simulink model "Casc_Filter_x4"  (Simulink 6.4)
settings: Solver=ode45  StartTime=0.0  StopTime=4100/sampling_freq  RelTol=1e-3
undefined symbols (not defined in the file): A, B, filter_clk, Fs, get, h_g, h_k, PCIN, sampling_freq
libraries: xbsIndex_r4 x851, dspsnks4 x9, simulink x2, dspsrcs4 x1
(part 8 of 8)

== system Casc_Filter_x4/DDC/DDC B/Gaussian FIR Filters/Gaussian FIR Filter1/Symmetric Data Flow/Symmetric Shift Register ==
  Shift In 1 : Inport
  Counter : Inport  Port=2
  Counter Inv : Inport  Port=3
  Shift In 2 : Inport  Port=4
  ASR : xbsIndex_r4/Addressable Shift Register  infer_latency=off  depth=12  initVector=[0]  en=off  dbl_ovrd=off  use_behavioral_HDL=off  use_rpm=off  block_type=addrsr
      settings: infoedit="Delay of  configurable length.  Any element  in the delay     line   can    be   addressed   and   driven    onto   the   output     port.<P><P>Hardware  notes: Implemented  using SRL16s.     If Virtex-4, Virtex-II or Spartan-3 devices are used, multiple SRLC16s are cascaded together."  xl_area=[9 0 0 18 0 0 0]  block_version=VER_STRING_GOES_HERE
  ASR1 : xbsIndex_r4/Addressable Shift Register  infer_latency=off  depth=12  initVector=[0]  en=off  dbl_ovrd=off  use_behavioral_HDL=off  use_rpm=off  block_type=addrsr
      settings: infoedit="Delay of  configurable length.  Any element  in the delay     line   can    be   addressed   and   driven    onto   the   output     port.<P><P>Hardware  notes: Implemented  using SRL16s.     If Virtex-4, Virtex-II or Spartan-3 devices are used, multiple SRLC16s are cascaded together."  xl_area=[9 0 0 18 0 0 0]  block_version=VER_STRING_GOES_HERE
  AddSub : xbsIndex_r4/AddSub  mode=Addition  use_carryin=off  use_carryout=off  en=off  latency=1  precision=User Defined  arith_type="Signed  (2's comp)"  n_bits=18  bin_pt=16  quantization="Round  (unbiased: +/- Inf)"  overflow=Saturate  dbl_ovrd=off  use_behavioral_HDL=off  pipelined=on  use_rpm=on  block_type=addsub
      settings: xl_area=[19 0 0 37 0 0 0]  block_version=VER_STRING_GOES_HERE
  Delay : xbsIndex_r4/Delay  en=off  latency=12  dbl_ovrd=off  reg_retiming=off  block_type=delay
      settings: infoedit=Hardware notes: A delay line is a chain, each link of which is an SRL16 followed by a flip-flop. If register retiming is enabled, the delay line is a chain of flip-flops.  xl_area=[9 18 0 18 0 0 0]  block_version=VER_STRING_GOES_HERE
  Delay1 : xbsIndex_r4/Delay  en=off  latency=12  dbl_ovrd=off  reg_retiming=off  block_type=delay
      settings: infoedit=Hardware notes: A delay line is a chain, each link of which is an SRL16 followed by a flip-flop. If register retiming is enabled, the delay line is a chain of flip-flops.  xl_area=[9 18 0 18 0 0 0]  block_version=VER_STRING_GOES_HERE
  Register : xbsIndex_r4/Register  init=0  rst=off  en=off  dbl_ovrd=off  block_type=register
      settings: block_version=8.2
  Register1 : xbsIndex_r4/Register  init=0  rst=off  en=off  dbl_ovrd=off  block_type=register
      settings: block_version=8.2
  Shift Out 1 : Outport
  Sum Out : Outport  Port=2
  Shift Out 2 : Outport  Port=3
  wires:
  Counter Inv/1 -> ASR1/2
  Shift In 1/1 -> ASR/1, Delay/1
  Shift In 2/1 -> Delay1/1, ASR1/1
  Counter/1 -> ASR/2
  ASR/1 -> Register/1
  ASR1/1 -> Register1/1
  AddSub/1 -> Sum Out/1
  Delay1/1 -> Shift Out 2/1
  Delay/1 -> Shift Out 1/1
  Register/1 -> AddSub/1
  Register1/1 -> AddSub/2

== system Casc_Filter_x4/DDC/DDC B/Gaussian FIR Filters/Gaussian FIR Filter1/Symmetric Data Flow/Symmetric Shift Register1 ==
  Shift In 1 : Inport
  Counter : Inport  Port=2
  Counter Inv : Inport  Port=3
  Shift In 2 : Inport  Port=4
  ASR : xbsIndex_r4/Addressable Shift Register  infer_latency=off  depth=12  initVector=[0]  en=off  dbl_ovrd=off  use_behavioral_HDL=off  use_rpm=off  block_type=addrsr
      settings: infoedit="Delay of  configurable length.  Any element  in the delay     line   can    be   addressed   and   driven    onto   the   output     port.<P><P>Hardware  notes: Implemented  using SRL16s.     If Virtex-4, Virtex-II or Spartan-3 devices are used, multiple SRLC16s are cascaded together."  xl_area=[9 0 0 18 0 0 0]  block_version=VER_STRING_GOES_HERE
  ASR1 : xbsIndex_r4/Addressable Shift Register  infer_latency=off  depth=12  initVector=[0]  en=off  dbl_ovrd=off  use_behavioral_HDL=off  use_rpm=off  block_type=addrsr
      settings: infoedit="Delay of  configurable length.  Any element  in the delay     line   can    be   addressed   and   driven    onto   the   output     port.<P><P>Hardware  notes: Implemented  using SRL16s.     If Virtex-4, Virtex-II or Spartan-3 devices are used, multiple SRLC16s are cascaded together."  xl_area=[9 0 0 18 0 0 0]  block_version=VER_STRING_GOES_HERE
  AddSub : xbsIndex_r4/AddSub  mode=Addition  use_carryin=off  use_carryout=off  en=off  latency=1  precision=User Defined  arith_type="Signed  (2's comp)"  n_bits=18  bin_pt=16  quantization="Round  (unbiased: +/- Inf)"  overflow=Saturate  dbl_ovrd=off  use_behavioral_HDL=off  pipelined=on  use_rpm=on  block_type=addsub
      settings: xl_area=[19 0 0 37 0 0 0]  block_version=VER_STRING_GOES_HERE
  Delay : xbsIndex_r4/Delay  en=off  latency=12  dbl_ovrd=off  reg_retiming=off  block_type=delay
      settings: infoedit=Hardware notes: A delay line is a chain, each link of which is an SRL16 followed by a flip-flop. If register retiming is enabled, the delay line is a chain of flip-flops.  xl_area=[9 18 0 18 0 0 0]  block_version=VER_STRING_GOES_HERE
  Delay1 : xbsIndex_r4/Delay  en=off  latency=12  dbl_ovrd=off  reg_retiming=off  block_type=delay
      settings: infoedit=Hardware notes: A delay line is a chain, each link of which is an SRL16 followed by a flip-flop. If register retiming is enabled, the delay line is a chain of flip-flops.  xl_area=[9 18 0 18 0 0 0]  block_version=VER_STRING_GOES_HERE
  Register : xbsIndex_r4/Register  init=0  rst=off  en=off  dbl_ovrd=off  block_type=register
      settings: block_version=8.2
  Register1 : xbsIndex_r4/Register  init=0  rst=off  en=off  dbl_ovrd=off  block_type=register
      settings: block_version=8.2
  Shift Out 1 : Outport
  Sum Out : Outport  Port=2
  Shift Out 2 : Outport  Port=3
  wires:
  Counter Inv/1 -> ASR1/2
  Shift In 1/1 -> ASR/1, Delay/1
  Shift In 2/1 -> Delay1/1, ASR1/1
  Counter/1 -> ASR/2
  ASR/1 -> Register/1
  ASR1/1 -> Register1/1
  AddSub/1 -> Sum Out/1
  Delay1/1 -> Shift Out 2/1
  Delay/1 -> Shift Out 1/1
  Register/1 -> AddSub/1
  Register1/1 -> AddSub/2

== system Casc_Filter_x4/DDC/DDC B/Gaussian FIR Filters/Gaussian FIR Filter1/Symmetric Data Flow/Symmetric Shift Register2 ==
  Shift In 1 : Inport
  Counter : Inport  Port=2
  Counter Inv : Inport  Port=3
  Shift In 2 : Inport  Port=4
  ASR : xbsIndex_r4/Addressable Shift Register  infer_latency=off  depth=12  initVector=[0]  en=off  dbl_ovrd=off  use_behavioral_HDL=off  use_rpm=off  block_type=addrsr
      settings: infoedit="Delay of  configurable length.  Any element  in the delay     line   can    be   addressed   and   driven    onto   the   output     port.<P><P>Hardware  notes: Implemented  using SRL16s.     If Virtex-4, Virtex-II or Spartan-3 devices are used, multiple SRLC16s are cascaded together."  xl_area=[9 0 0 18 0 0 0]  block_version=VER_STRING_GOES_HERE
  ASR1 : xbsIndex_r4/Addressable Shift Register  infer_latency=off  depth=12  initVector=[0]  en=off  dbl_ovrd=off  use_behavioral_HDL=off  use_rpm=off  block_type=addrsr
      settings: infoedit="Delay of  configurable length.  Any element  in the delay     line   can    be   addressed   and   driven    onto   the   output     port.<P><P>Hardware  notes: Implemented  using SRL16s.     If Virtex-4, Virtex-II or Spartan-3 devices are used, multiple SRLC16s are cascaded together."  xl_area=[9 0 0 18 0 0 0]  block_version=VER_STRING_GOES_HERE
  AddSub : xbsIndex_r4/AddSub  mode=Addition  use_carryin=off  use_carryout=off  en=off  latency=1  precision=User Defined  arith_type="Signed  (2's comp)"  n_bits=18  bin_pt=16  quantization="Round  (unbiased: +/- Inf)"  overflow=Saturate  dbl_ovrd=off  use_behavioral_HDL=off  pipelined=on  use_rpm=on  block_type=addsub
      settings: xl_area=[19 0 0 37 0 0 0]  block_version=VER_STRING_GOES_HERE
  Delay : xbsIndex_r4/Delay  en=off  latency=12  dbl_ovrd=off  reg_retiming=off  block_type=delay
      settings: infoedit=Hardware notes: A delay line is a chain, each link of which is an SRL16 followed by a flip-flop. If register retiming is enabled, the delay line is a chain of flip-flops.  xl_area=[9 18 0 18 0 0 0]  block_version=VER_STRING_GOES_HERE
  Delay1 : xbsIndex_r4/Delay  en=off  latency=12  dbl_ovrd=off  reg_retiming=off  block_type=delay
      settings: infoedit=Hardware notes: A delay line is a chain, each link of which is an SRL16 followed by a flip-flop. If register retiming is enabled, the delay line is a chain of flip-flops.  xl_area=[9 18 0 18 0 0 0]  block_version=VER_STRING_GOES_HERE
  Register : xbsIndex_r4/Register  init=0  rst=off  en=off  dbl_ovrd=off  block_type=register
      settings: block_version=8.2
  Register1 : xbsIndex_r4/Register  init=0  rst=off  en=off  dbl_ovrd=off  block_type=register
      settings: block_version=8.2
  Shift Out 1 : Outport
  Sum Out : Outport  Port=2
  Shift Out 2 : Outport  Port=3
  wires:
  Counter Inv/1 -> ASR1/2
  Shift In 1/1 -> ASR/1, Delay/1
  Shift In 2/1 -> Delay1/1, ASR1/1
  Counter/1 -> ASR/2
  ASR/1 -> Register/1
  ASR1/1 -> Register1/1
  AddSub/1 -> Sum Out/1
  Delay1/1 -> Shift Out 2/1
  Delay/1 -> Shift Out 1/1
  Register/1 -> AddSub/1
  Register1/1 -> AddSub/2

== system Casc_Filter_x4/DDC/DDC C/Gaussian FIR Filters/Gaussian FIR Filter/Symmetric Data Flow/Symmetric Shift Register ==
  Shift In 1 : Inport
  Counter : Inport  Port=2
  Counter Inv : Inport  Port=3
  Shift In 2 : Inport  Port=4
  ASR : xbsIndex_r4/Addressable Shift Register  infer_latency=off  depth=12  initVector=[0]  en=off  dbl_ovrd=off  use_behavioral_HDL=off  use_rpm=off  block_type=addrsr
      settings: infoedit="Delay of  configurable length.  Any element  in the delay     line   can    be   addressed   and   driven    onto   the   output     port.<P><P>Hardware  notes: Implemented  using SRL16s.     If Virtex-4, Virtex-II or Spartan-3 devices are used, multiple SRLC16s are cascaded together."  xl_area=[9 0 0 18 0 0 0]  block_version=VER_STRING_GOES_HERE
  ASR1 : xbsIndex_r4/Addressable Shift Register  infer_latency=off  depth=12  initVector=[0]  en=off  dbl_ovrd=off  use_behavioral_HDL=off  use_rpm=off  block_type=addrsr
      settings: infoedit="Delay of  configurable length.  Any element  in the delay     line   can    be   addressed   and   driven    onto   the   output     port.<P><P>Hardware  notes: Implemented  using SRL16s.     If Virtex-4, Virtex-II or Spartan-3 devices are used, multiple SRLC16s are cascaded together."  xl_area=[9 0 0 18 0 0 0]  block_version=VER_STRING_GOES_HERE
  AddSub : xbsIndex_r4/AddSub  mode=Addition  use_carryin=off  use_carryout=off  en=off  latency=1  precision=User Defined  arith_type="Signed  (2's comp)"  n_bits=18  bin_pt=16  quantization="Round  (unbiased: +/- Inf)"  overflow=Saturate  dbl_ovrd=off  use_behavioral_HDL=off  pipelined=on  use_rpm=on  block_type=addsub
      settings: xl_area=[19 0 0 37 0 0 0]  block_version=VER_STRING_GOES_HERE
  Delay : xbsIndex_r4/Delay  en=off  latency=12  dbl_ovrd=off  reg_retiming=off  block_type=delay
      settings: infoedit=Hardware notes: A delay line is a chain, each link of which is an SRL16 followed by a flip-flop. If register retiming is enabled, the delay line is a chain of flip-flops.  xl_area=[9 18 0 18 0 0 0]  block_version=VER_STRING_GOES_HERE
  Delay1 : xbsIndex_r4/Delay  en=off  latency=12  dbl_ovrd=off  reg_retiming=off  block_type=delay
      settings: infoedit=Hardware notes: A delay line is a chain, each link of which is an SRL16 followed by a flip-flop. If register retiming is enabled, the delay line is a chain of flip-flops.  xl_area=[9 18 0 18 0 0 0]  block_version=VER_STRING_GOES_HERE
  Register : xbsIndex_r4/Register  init=0  rst=off  en=off  dbl_ovrd=off  block_type=register
      settings: block_version=8.2
  Register1 : xbsIndex_r4/Register  init=0  rst=off  en=off  dbl_ovrd=off  block_type=register
      settings: block_version=8.2
  Shift Out 1 : Outport
  Sum Out : Outport  Port=2
  Shift Out 2 : Outport  Port=3
  wires:
  Counter Inv/1 -> ASR1/2
  Shift In 1/1 -> ASR/1, Delay/1
  Shift In 2/1 -> Delay1/1, ASR1/1
  Counter/1 -> ASR/2
  ASR/1 -> Register/1
  ASR1/1 -> Register1/1
  AddSub/1 -> Sum Out/1
  Delay1/1 -> Shift Out 2/1
  Delay/1 -> Shift Out 1/1
  Register/1 -> AddSub/1
  Register1/1 -> AddSub/2

== system Casc_Filter_x4/DDC/DDC C/Gaussian FIR Filters/Gaussian FIR Filter/Symmetric Data Flow/Symmetric Shift Register1 ==
  Shift In 1 : Inport
  Counter : Inport  Port=2
  Counter Inv : Inport  Port=3
  Shift In 2 : Inport  Port=4
  ASR : xbsIndex_r4/Addressable Shift Register  infer_latency=off  depth=12  initVector=[0]  en=off  dbl_ovrd=off  use_behavioral_HDL=off  use_rpm=off  block_type=addrsr
      settings: infoedit="Delay of  configurable length.  Any element  in the delay     line   can    be   addressed   and   driven    onto   the   output     port.<P><P>Hardware  notes: Implemented  using SRL16s.     If Virtex-4, Virtex-II or Spartan-3 devices are used, multiple SRLC16s are cascaded together."  xl_area=[9 0 0 18 0 0 0]  block_version=VER_STRING_GOES_HERE
  ASR1 : xbsIndex_r4/Addressable Shift Register  infer_latency=off  depth=12  initVector=[0]  en=off  dbl_ovrd=off  use_behavioral_HDL=off  use_rpm=off  block_type=addrsr
      settings: infoedit="Delay of  configurable length.  Any element  in the delay     line   can    be   addressed   and   driven    onto   the   output     port.<P><P>Hardware  notes: Implemented  using SRL16s.     If Virtex-4, Virtex-II or Spartan-3 devices are used, multiple SRLC16s are cascaded together."  xl_area=[9 0 0 18 0 0 0]  block_version=VER_STRING_GOES_HERE
  AddSub : xbsIndex_r4/AddSub  mode=Addition  use_carryin=off  use_carryout=off  en=off  latency=1  precision=User Defined  arith_type="Signed  (2's comp)"  n_bits=18  bin_pt=16  quantization="Round  (unbiased: +/- Inf)"  overflow=Saturate  dbl_ovrd=off  use_behavioral_HDL=off  pipelined=on  use_rpm=on  block_type=addsub
      settings: xl_area=[19 0 0 37 0 0 0]  block_version=VER_STRING_GOES_HERE
  Delay : xbsIndex_r4/Delay  en=off  latency=12  dbl_ovrd=off  reg_retiming=off  block_type=delay
      settings: infoedit=Hardware notes: A delay line is a chain, each link of which is an SRL16 followed by a flip-flop. If register retiming is enabled, the delay line is a chain of flip-flops.  xl_area=[9 18 0 18 0 0 0]  block_version=VER_STRING_GOES_HERE
  Delay1 : xbsIndex_r4/Delay  en=off  latency=12  dbl_ovrd=off  reg_retiming=off  block_type=delay
      settings: infoedit=Hardware notes: A delay line is a chain, each link of which is an SRL16 followed by a flip-flop. If register retiming is enabled, the delay line is a chain of flip-flops.  xl_area=[9 18 0 18 0 0 0]  block_version=VER_STRING_GOES_HERE
  Register : xbsIndex_r4/Register  init=0  rst=off  en=off  dbl_ovrd=off  block_type=register
      settings: block_version=8.2
  Register1 : xbsIndex_r4/Register  init=0  rst=off  en=off  dbl_ovrd=off  block_type=register
      settings: block_version=8.2
  Shift Out 1 : Outport
  Sum Out : Outport  Port=2
  Shift Out 2 : Outport  Port=3
  wires:
  Counter Inv/1 -> ASR1/2
  Shift In 1/1 -> ASR/1, Delay/1
  Shift In 2/1 -> Delay1/1, ASR1/1
  Counter/1 -> ASR/2
  ASR/1 -> Register/1
  ASR1/1 -> Register1/1
  AddSub/1 -> Sum Out/1
  Delay1/1 -> Shift Out 2/1
  Delay/1 -> Shift Out 1/1
  Register/1 -> AddSub/1
  Register1/1 -> AddSub/2

== system Casc_Filter_x4/DDC/DDC C/Gaussian FIR Filters/Gaussian FIR Filter/Symmetric Data Flow/Symmetric Shift Register2 ==
  Shift In 1 : Inport
  Counter : Inport  Port=2
  Counter Inv : Inport  Port=3
  Shift In 2 : Inport  Port=4
  ASR : xbsIndex_r4/Addressable Shift Register  infer_latency=off  depth=12  initVector=[0]  en=off  dbl_ovrd=off  use_behavioral_HDL=off  use_rpm=off  block_type=addrsr
      settings: infoedit="Delay of  configurable length.  Any element  in the delay     line   can    be   addressed   and   driven    onto   the   output     port.<P><P>Hardware  notes: Implemented  using SRL16s.     If Virtex-4, Virtex-II or Spartan-3 devices are used, multiple SRLC16s are cascaded together."  xl_area=[9 0 0 18 0 0 0]  block_version=VER_STRING_GOES_HERE
  ASR1 : xbsIndex_r4/Addressable Shift Register  infer_latency=off  depth=12  initVector=[0]  en=off  dbl_ovrd=off  use_behavioral_HDL=off  use_rpm=off  block_type=addrsr
      settings: infoedit="Delay of  configurable length.  Any element  in the delay     line   can    be   addressed   and   driven    onto   the   output     port.<P><P>Hardware  notes: Implemented  using SRL16s.     If Virtex-4, Virtex-II or Spartan-3 devices are used, multiple SRLC16s are cascaded together."  xl_area=[9 0 0 18 0 0 0]  block_version=VER_STRING_GOES_HERE
  AddSub : xbsIndex_r4/AddSub  mode=Addition  use_carryin=off  use_carryout=off  en=off  latency=1  precision=User Defined  arith_type="Signed  (2's comp)"  n_bits=18  bin_pt=16  quantization="Round  (unbiased: +/- Inf)"  overflow=Saturate  dbl_ovrd=off  use_behavioral_HDL=off  pipelined=on  use_rpm=on  block_type=addsub
      settings: xl_area=[19 0 0 37 0 0 0]  block_version=VER_STRING_GOES_HERE
  Delay : xbsIndex_r4/Delay  en=off  latency=12  dbl_ovrd=off  reg_retiming=off  block_type=delay
      settings: infoedit=Hardware notes: A delay line is a chain, each link of which is an SRL16 followed by a flip-flop. If register retiming is enabled, the delay line is a chain of flip-flops.  xl_area=[9 18 0 18 0 0 0]  block_version=VER_STRING_GOES_HERE
  Delay1 : xbsIndex_r4/Delay  en=off  latency=12  dbl_ovrd=off  reg_retiming=off  block_type=delay
      settings: infoedit=Hardware notes: A delay line is a chain, each link of which is an SRL16 followed by a flip-flop. If register retiming is enabled, the delay line is a chain of flip-flops.  xl_area=[9 18 0 18 0 0 0]  block_version=VER_STRING_GOES_HERE
  Register : xbsIndex_r4/Register  init=0  rst=off  en=off  dbl_ovrd=off  block_type=register
      settings: block_version=8.2
  Register1 : xbsIndex_r4/Register  init=0  rst=off  en=off  dbl_ovrd=off  block_type=register
      settings: block_version=8.2
  Shift Out 1 : Outport
  Sum Out : Outport  Port=2
  Shift Out 2 : Outport  Port=3
  wires:
  Counter Inv/1 -> ASR1/2
  Shift In 1/1 -> ASR/1, Delay/1
  Shift In 2/1 -> Delay1/1, ASR1/1
  Counter/1 -> ASR/2
  ASR/1 -> Register/1
  ASR1/1 -> Register1/1
  AddSub/1 -> Sum Out/1
  Delay1/1 -> Shift Out 2/1
  Delay/1 -> Shift Out 1/1
  Register/1 -> AddSub/1
  Register1/1 -> AddSub/2

== system Casc_Filter_x4/DDC/DDC C/Gaussian FIR Filters/Gaussian FIR Filter1/Symmetric Data Flow/Symmetric Shift Register ==
  Shift In 1 : Inport
  Counter : Inport  Port=2
  Counter Inv : Inport  Port=3
  Shift In 2 : Inport  Port=4
  ASR : xbsIndex_r4/Addressable Shift Register  infer_latency=off  depth=12  initVector=[0]  en=off  dbl_ovrd=off  use_behavioral_HDL=off  use_rpm=off  block_type=addrsr
      settings: infoedit="Delay of  configurable length.  Any element  in the delay     line   can    be   addressed   and   driven    onto   the   output     port.<P><P>Hardware  notes: Implemented  using SRL16s.     If Virtex-4, Virtex-II or Spartan-3 devices are used, multiple SRLC16s are cascaded together."  xl_area=[9 0 0 18 0 0 0]  block_version=VER_STRING_GOES_HERE
  ASR1 : xbsIndex_r4/Addressable Shift Register  infer_latency=off  depth=12  initVector=[0]  en=off  dbl_ovrd=off  use_behavioral_HDL=off  use_rpm=off  block_type=addrsr
      settings: infoedit="Delay of  configurable length.  Any element  in the delay     line   can    be   addressed   and   driven    onto   the   output     port.<P><P>Hardware  notes: Implemented  using SRL16s.     If Virtex-4, Virtex-II or Spartan-3 devices are used, multiple SRLC16s are cascaded together."  xl_area=[9 0 0 18 0 0 0]  block_version=VER_STRING_GOES_HERE
  AddSub : xbsIndex_r4/AddSub  mode=Addition  use_carryin=off  use_carryout=off  en=off  latency=1  precision=User Defined  arith_type="Signed  (2's comp)"  n_bits=18  bin_pt=16  quantization="Round  (unbiased: +/- Inf)"  overflow=Saturate  dbl_ovrd=off  use_behavioral_HDL=off  pipelined=on  use_rpm=on  block_type=addsub
      settings: xl_area=[19 0 0 37 0 0 0]  block_version=VER_STRING_GOES_HERE
  Delay : xbsIndex_r4/Delay  en=off  latency=12  dbl_ovrd=off  reg_retiming=off  block_type=delay
      settings: infoedit=Hardware notes: A delay line is a chain, each link of which is an SRL16 followed by a flip-flop. If register retiming is enabled, the delay line is a chain of flip-flops.  xl_area=[9 18 0 18 0 0 0]  block_version=VER_STRING_GOES_HERE
  Delay1 : xbsIndex_r4/Delay  en=off  latency=12  dbl_ovrd=off  reg_retiming=off  block_type=delay
      settings: infoedit=Hardware notes: A delay line is a chain, each link of which is an SRL16 followed by a flip-flop. If register retiming is enabled, the delay line is a chain of flip-flops.  xl_area=[9 18 0 18 0 0 0]  block_version=VER_STRING_GOES_HERE
  Register : xbsIndex_r4/Register  init=0  rst=off  en=off  dbl_ovrd=off  block_type=register
      settings: block_version=8.2
  Register1 : xbsIndex_r4/Register  init=0  rst=off  en=off  dbl_ovrd=off  block_type=register
      settings: block_version=8.2
  Shift Out 1 : Outport
  Sum Out : Outport  Port=2
  Shift Out 2 : Outport  Port=3
  wires:
  Counter Inv/1 -> ASR1/2
  Shift In 1/1 -> ASR/1, Delay/1
  Shift In 2/1 -> Delay1/1, ASR1/1
  Counter/1 -> ASR/2
  ASR/1 -> Register/1
  ASR1/1 -> Register1/1
  AddSub/1 -> Sum Out/1
  Delay1/1 -> Shift Out 2/1
  Delay/1 -> Shift Out 1/1
  Register/1 -> AddSub/1
  Register1/1 -> AddSub/2

== system Casc_Filter_x4/DDC/DDC C/Gaussian FIR Filters/Gaussian FIR Filter1/Symmetric Data Flow/Symmetric Shift Register1 ==
  Shift In 1 : Inport
  Counter : Inport  Port=2
  Counter Inv : Inport  Port=3
  Shift In 2 : Inport  Port=4
  ASR : xbsIndex_r4/Addressable Shift Register  infer_latency=off  depth=12  initVector=[0]  en=off  dbl_ovrd=off  use_behavioral_HDL=off  use_rpm=off  block_type=addrsr
      settings: infoedit="Delay of  configurable length.  Any element  in the delay     line   can    be   addressed   and   driven    onto   the   output     port.<P><P>Hardware  notes: Implemented  using SRL16s.     If Virtex-4, Virtex-II or Spartan-3 devices are used, multiple SRLC16s are cascaded together."  xl_area=[9 0 0 18 0 0 0]  block_version=VER_STRING_GOES_HERE
  ASR1 : xbsIndex_r4/Addressable Shift Register  infer_latency=off  depth=12  initVector=[0]  en=off  dbl_ovrd=off  use_behavioral_HDL=off  use_rpm=off  block_type=addrsr
      settings: infoedit="Delay of  configurable length.  Any element  in the delay     line   can    be   addressed   and   driven    onto   the   output     port.<P><P>Hardware  notes: Implemented  using SRL16s.     If Virtex-4, Virtex-II or Spartan-3 devices are used, multiple SRLC16s are cascaded together."  xl_area=[9 0 0 18 0 0 0]  block_version=VER_STRING_GOES_HERE
  AddSub : xbsIndex_r4/AddSub  mode=Addition  use_carryin=off  use_carryout=off  en=off  latency=1  precision=User Defined  arith_type="Signed  (2's comp)"  n_bits=18  bin_pt=16  quantization="Round  (unbiased: +/- Inf)"  overflow=Saturate  dbl_ovrd=off  use_behavioral_HDL=off  pipelined=on  use_rpm=on  block_type=addsub
      settings: xl_area=[19 0 0 37 0 0 0]  block_version=VER_STRING_GOES_HERE
  Delay : xbsIndex_r4/Delay  en=off  latency=12  dbl_ovrd=off  reg_retiming=off  block_type=delay
      settings: infoedit=Hardware notes: A delay line is a chain, each link of which is an SRL16 followed by a flip-flop. If register retiming is enabled, the delay line is a chain of flip-flops.  xl_area=[9 18 0 18 0 0 0]  block_version=VER_STRING_GOES_HERE
  Delay1 : xbsIndex_r4/Delay  en=off  latency=12  dbl_ovrd=off  reg_retiming=off  block_type=delay
      settings: infoedit=Hardware notes: A delay line is a chain, each link of which is an SRL16 followed by a flip-flop. If register retiming is enabled, the delay line is a chain of flip-flops.  xl_area=[9 18 0 18 0 0 0]  block_version=VER_STRING_GOES_HERE
  Register : xbsIndex_r4/Register  init=0  rst=off  en=off  dbl_ovrd=off  block_type=register
      settings: block_version=8.2
  Register1 : xbsIndex_r4/Register  init=0  rst=off  en=off  dbl_ovrd=off  block_type=register
      settings: block_version=8.2
  Shift Out 1 : Outport
  Sum Out : Outport  Port=2
  Shift Out 2 : Outport  Port=3
  wires:
  Counter Inv/1 -> ASR1/2
  Shift In 1/1 -> ASR/1, Delay/1
  Shift In 2/1 -> Delay1/1, ASR1/1
  Counter/1 -> ASR/2
  ASR/1 -> Register/1
  ASR1/1 -> Register1/1
  AddSub/1 -> Sum Out/1
  Delay1/1 -> Shift Out 2/1
  Delay/1 -> Shift Out 1/1
  Register/1 -> AddSub/1
  Register1/1 -> AddSub/2

== system Casc_Filter_x4/DDC/DDC C/Gaussian FIR Filters/Gaussian FIR Filter1/Symmetric Data Flow/Symmetric Shift Register2 ==
  Shift In 1 : Inport
  Counter : Inport  Port=2
  Counter Inv : Inport  Port=3
  Shift In 2 : Inport  Port=4
  ASR : xbsIndex_r4/Addressable Shift Register  infer_latency=off  depth=12  initVector=[0]  en=off  dbl_ovrd=off  use_behavioral_HDL=off  use_rpm=off  block_type=addrsr
      settings: infoedit="Delay of  configurable length.  Any element  in the delay     line   can    be   addressed   and   driven    onto   the   output     port.<P><P>Hardware  notes: Implemented  using SRL16s.     If Virtex-4, Virtex-II or Spartan-3 devices are used, multiple SRLC16s are cascaded together."  xl_area=[9 0 0 18 0 0 0]  block_version=VER_STRING_GOES_HERE
  ASR1 : xbsIndex_r4/Addressable Shift Register  infer_latency=off  depth=12  initVector=[0]  en=off  dbl_ovrd=off  use_behavioral_HDL=off  use_rpm=off  block_type=addrsr
      settings: infoedit="Delay of  configurable length.  Any element  in the delay     line   can    be   addressed   and   driven    onto   the   output     port.<P><P>Hardware  notes: Implemented  using SRL16s.     If Virtex-4, Virtex-II or Spartan-3 devices are used, multiple SRLC16s are cascaded together."  xl_area=[9 0 0 18 0 0 0]  block_version=VER_STRING_GOES_HERE
  AddSub : xbsIndex_r4/AddSub  mode=Addition  use_carryin=off  use_carryout=off  en=off  latency=1  precision=User Defined  arith_type="Signed  (2's comp)"  n_bits=18  bin_pt=16  quantization="Round  (unbiased: +/- Inf)"  overflow=Saturate  dbl_ovrd=off  use_behavioral_HDL=off  pipelined=on  use_rpm=on  block_type=addsub
      settings: xl_area=[19 0 0 37 0 0 0]  block_version=VER_STRING_GOES_HERE
  Delay : xbsIndex_r4/Delay  en=off  latency=12  dbl_ovrd=off  reg_retiming=off  block_type=delay
      settings: infoedit=Hardware notes: A delay line is a chain, each link of which is an SRL16 followed by a flip-flop. If register retiming is enabled, the delay line is a chain of flip-flops.  xl_area=[9 18 0 18 0 0 0]  block_version=VER_STRING_GOES_HERE
  Delay1 : xbsIndex_r4/Delay  en=off  latency=12  dbl_ovrd=off  reg_retiming=off  block_type=delay
      settings: infoedit=Hardware notes: A delay line is a chain, each link of which is an SRL16 followed by a flip-flop. If register retiming is enabled, the delay line is a chain of flip-flops.  xl_area=[9 18 0 18 0 0 0]  block_version=VER_STRING_GOES_HERE
  Register : xbsIndex_r4/Register  init=0  rst=off  en=off  dbl_ovrd=off  block_type=register
      settings: block_version=8.2
  Register1 : xbsIndex_r4/Register  init=0  rst=off  en=off  dbl_ovrd=off  block_type=register
      settings: block_version=8.2
  Shift Out 1 : Outport
  Sum Out : Outport  Port=2
  Shift Out 2 : Outport  Port=3
  wires:
  Counter Inv/1 -> ASR1/2
  Shift In 1/1 -> ASR/1, Delay/1
  Shift In 2/1 -> Delay1/1, ASR1/1
  Counter/1 -> ASR/2
  ASR/1 -> Register/1
  ASR1/1 -> Register1/1
  AddSub/1 -> Sum Out/1
  Delay1/1 -> Shift Out 2/1
  Delay/1 -> Shift Out 1/1
  Register/1 -> AddSub/1
  Register1/1 -> AddSub/2

== system Casc_Filter_x4/DDC/DDC D/Gaussian FIR Filters/Gaussian FIR Filter/Symmetric Data Flow/Symmetric Shift Register ==
  Shift In 1 : Inport
  Counter : Inport  Port=2
  Counter Inv : Inport  Port=3
  Shift In 2 : Inport  Port=4
  ASR : xbsIndex_r4/Addressable Shift Register  infer_latency=off  depth=12  initVector=[0]  en=off  dbl_ovrd=off  use_behavioral_HDL=off  use_rpm=off  block_type=addrsr
      settings: infoedit="Delay of  configurable length.  Any element  in the delay     line   can    be   addressed   and   driven    onto   the   output     port.<P><P>Hardware  notes: Implemented  using SRL16s.     If Virtex-4, Virtex-II or Spartan-3 devices are used, multiple SRLC16s are cascaded together."  xl_area=[9 0 0 18 0 0 0]  block_version=VER_STRING_GOES_HERE
  ASR1 : xbsIndex_r4/Addressable Shift Register  infer_latency=off  depth=12  initVector=[0]  en=off  dbl_ovrd=off  use_behavioral_HDL=off  use_rpm=off  block_type=addrsr
      settings: infoedit="Delay of  configurable length.  Any element  in the delay     line   can    be   addressed   and   driven    onto   the   output     port.<P><P>Hardware  notes: Implemented  using SRL16s.     If Virtex-4, Virtex-II or Spartan-3 devices are used, multiple SRLC16s are cascaded together."  xl_area=[9 0 0 18 0 0 0]  block_version=VER_STRING_GOES_HERE
  AddSub : xbsIndex_r4/AddSub  mode=Addition  use_carryin=off  use_carryout=off  en=off  latency=1  precision=User Defined  arith_type="Signed  (2's comp)"  n_bits=18  bin_pt=16  quantization="Round  (unbiased: +/- Inf)"  overflow=Saturate  dbl_ovrd=off  use_behavioral_HDL=off  pipelined=on  use_rpm=on  block_type=addsub
      settings: xl_area=[19 0 0 37 0 0 0]  block_version=VER_STRING_GOES_HERE
  Delay : xbsIndex_r4/Delay  en=off  latency=12  dbl_ovrd=off  reg_retiming=off  block_type=delay
      settings: infoedit=Hardware notes: A delay line is a chain, each link of which is an SRL16 followed by a flip-flop. If register retiming is enabled, the delay line is a chain of flip-flops.  xl_area=[9 18 0 18 0 0 0]  block_version=VER_STRING_GOES_HERE
  Delay1 : xbsIndex_r4/Delay  en=off  latency=12  dbl_ovrd=off  reg_retiming=off  block_type=delay
      settings: infoedit=Hardware notes: A delay line is a chain, each link of which is an SRL16 followed by a flip-flop. If register retiming is enabled, the delay line is a chain of flip-flops.  xl_area=[9 18 0 18 0 0 0]  block_version=VER_STRING_GOES_HERE
  Register : xbsIndex_r4/Register  init=0  rst=off  en=off  dbl_ovrd=off  block_type=register
      settings: block_version=8.2
  Register1 : xbsIndex_r4/Register  init=0  rst=off  en=off  dbl_ovrd=off  block_type=register
      settings: block_version=8.2
  Shift Out 1 : Outport
  Sum Out : Outport  Port=2
  Shift Out 2 : Outport  Port=3
  wires:
  Counter Inv/1 -> ASR1/2
  Shift In 1/1 -> ASR/1, Delay/1
  Shift In 2/1 -> Delay1/1, ASR1/1
  Counter/1 -> ASR/2
  ASR/1 -> Register/1
  ASR1/1 -> Register1/1
  AddSub/1 -> Sum Out/1
  Delay1/1 -> Shift Out 2/1
  Delay/1 -> Shift Out 1/1
  Register/1 -> AddSub/1
  Register1/1 -> AddSub/2

== system Casc_Filter_x4/DDC/DDC D/Gaussian FIR Filters/Gaussian FIR Filter/Symmetric Data Flow/Symmetric Shift Register1 ==
  Shift In 1 : Inport
  Counter : Inport  Port=2
  Counter Inv : Inport  Port=3
  Shift In 2 : Inport  Port=4
  ASR : xbsIndex_r4/Addressable Shift Register  infer_latency=off  depth=12  initVector=[0]  en=off  dbl_ovrd=off  use_behavioral_HDL=off  use_rpm=off  block_type=addrsr
      settings: infoedit="Delay of  configurable length.  Any element  in the delay     line   can    be   addressed   and   driven    onto   the   output     port.<P><P>Hardware  notes: Implemented  using SRL16s.     If Virtex-4, Virtex-II or Spartan-3 devices are used, multiple SRLC16s are cascaded together."  xl_area=[9 0 0 18 0 0 0]  block_version=VER_STRING_GOES_HERE
  ASR1 : xbsIndex_r4/Addressable Shift Register  infer_latency=off  depth=12  initVector=[0]  en=off  dbl_ovrd=off  use_behavioral_HDL=off  use_rpm=off  block_type=addrsr
      settings: infoedit="Delay of  configurable length.  Any element  in the delay     line   can    be   addressed   and   driven    onto   the   output     port.<P><P>Hardware  notes: Implemented  using SRL16s.     If Virtex-4, Virtex-II or Spartan-3 devices are used, multiple SRLC16s are cascaded together."  xl_area=[9 0 0 18 0 0 0]  block_version=VER_STRING_GOES_HERE
  AddSub : xbsIndex_r4/AddSub  mode=Addition  use_carryin=off  use_carryout=off  en=off  latency=1  precision=User Defined  arith_type="Signed  (2's comp)"  n_bits=18  bin_pt=16  quantization="Round  (unbiased: +/- Inf)"  overflow=Saturate  dbl_ovrd=off  use_behavioral_HDL=off  pipelined=on  use_rpm=on  block_type=addsub
      settings: xl_area=[19 0 0 37 0 0 0]  block_version=VER_STRING_GOES_HERE
  Delay : xbsIndex_r4/Delay  en=off  latency=12  dbl_ovrd=off  reg_retiming=off  block_type=delay
      settings: infoedit=Hardware notes: A delay line is a chain, each link of which is an SRL16 followed by a flip-flop. If register retiming is enabled, the delay line is a chain of flip-flops.  xl_area=[9 18 0 18 0 0 0]  block_version=VER_STRING_GOES_HERE
  Delay1 : xbsIndex_r4/Delay  en=off  latency=12  dbl_ovrd=off  reg_retiming=off  block_type=delay
      settings: infoedit=Hardware notes: A delay line is a chain, each link of which is an SRL16 followed by a flip-flop. If register retiming is enabled, the delay line is a chain of flip-flops.  xl_area=[9 18 0 18 0 0 0]  block_version=VER_STRING_GOES_HERE
  Register : xbsIndex_r4/Register  init=0  rst=off  en=off  dbl_ovrd=off  block_type=register
      settings: block_version=8.2
  Register1 : xbsIndex_r4/Register  init=0  rst=off  en=off  dbl_ovrd=off  block_type=register
      settings: block_version=8.2
  Shift Out 1 : Outport
  Sum Out : Outport  Port=2
  Shift Out 2 : Outport  Port=3
  wires:
  Counter Inv/1 -> ASR1/2
  Shift In 1/1 -> ASR/1, Delay/1
  Shift In 2/1 -> Delay1/1, ASR1/1
  Counter/1 -> ASR/2
  ASR/1 -> Register/1
  ASR1/1 -> Register1/1
  AddSub/1 -> Sum Out/1
  Delay1/1 -> Shift Out 2/1
  Delay/1 -> Shift Out 1/1
  Register/1 -> AddSub/1
  Register1/1 -> AddSub/2

== system Casc_Filter_x4/DDC/DDC D/Gaussian FIR Filters/Gaussian FIR Filter/Symmetric Data Flow/Symmetric Shift Register2 ==
  Shift In 1 : Inport
  Counter : Inport  Port=2
  Counter Inv : Inport  Port=3
  Shift In 2 : Inport  Port=4
  ASR : xbsIndex_r4/Addressable Shift Register  infer_latency=off  depth=12  initVector=[0]  en=off  dbl_ovrd=off  use_behavioral_HDL=off  use_rpm=off  block_type=addrsr
      settings: infoedit="Delay of  configurable length.  Any element  in the delay     line   can    be   addressed   and   driven    onto   the   output     port.<P><P>Hardware  notes: Implemented  using SRL16s.     If Virtex-4, Virtex-II or Spartan-3 devices are used, multiple SRLC16s are cascaded together."  xl_area=[9 0 0 18 0 0 0]  block_version=VER_STRING_GOES_HERE
  ASR1 : xbsIndex_r4/Addressable Shift Register  infer_latency=off  depth=12  initVector=[0]  en=off  dbl_ovrd=off  use_behavioral_HDL=off  use_rpm=off  block_type=addrsr
      settings: infoedit="Delay of  configurable length.  Any element  in the delay     line   can    be   addressed   and   driven    onto   the   output     port.<P><P>Hardware  notes: Implemented  using SRL16s.     If Virtex-4, Virtex-II or Spartan-3 devices are used, multiple SRLC16s are cascaded together."  xl_area=[9 0 0 18 0 0 0]  block_version=VER_STRING_GOES_HERE
  AddSub : xbsIndex_r4/AddSub  mode=Addition  use_carryin=off  use_carryout=off  en=off  latency=1  precision=User Defined  arith_type="Signed  (2's comp)"  n_bits=18  bin_pt=16  quantization="Round  (unbiased: +/- Inf)"  overflow=Saturate  dbl_ovrd=off  use_behavioral_HDL=off  pipelined=on  use_rpm=on  block_type=addsub
      settings: xl_area=[19 0 0 37 0 0 0]  block_version=VER_STRING_GOES_HERE
  Delay : xbsIndex_r4/Delay  en=off  latency=12  dbl_ovrd=off  reg_retiming=off  block_type=delay
      settings: infoedit=Hardware notes: A delay line is a chain, each link of which is an SRL16 followed by a flip-flop. If register retiming is enabled, the delay line is a chain of flip-flops.  xl_area=[9 18 0 18 0 0 0]  block_version=VER_STRING_GOES_HERE
  Delay1 : xbsIndex_r4/Delay  en=off  latency=12  dbl_ovrd=off  reg_retiming=off  block_type=delay
      settings: infoedit=Hardware notes: A delay line is a chain, each link of which is an SRL16 followed by a flip-flop. If register retiming is enabled, the delay line is a chain of flip-flops.  xl_area=[9 18 0 18 0 0 0]  block_version=VER_STRING_GOES_HERE
  Register : xbsIndex_r4/Register  init=0  rst=off  en=off  dbl_ovrd=off  block_type=register
      settings: block_version=8.2
  Register1 : xbsIndex_r4/Register  init=0  rst=off  en=off  dbl_ovrd=off  block_type=register
      settings: block_version=8.2
  Shift Out 1 : Outport
  Sum Out : Outport  Port=2
  Shift Out 2 : Outport  Port=3
  wires:
  Counter Inv/1 -> ASR1/2
  Shift In 1/1 -> ASR/1, Delay/1
  Shift In 2/1 -> Delay1/1, ASR1/1
  Counter/1 -> ASR/2
  ASR/1 -> Register/1
  ASR1/1 -> Register1/1
  AddSub/1 -> Sum Out/1
  Delay1/1 -> Shift Out 2/1
  Delay/1 -> Shift Out 1/1
  Register/1 -> AddSub/1
  Register1/1 -> AddSub/2

== system Casc_Filter_x4/DDC/DDC D/Gaussian FIR Filters/Gaussian FIR Filter1/Symmetric Data Flow/Symmetric Shift Register ==
  Shift In 1 : Inport
  Counter : Inport  Port=2
  Counter Inv : Inport  Port=3
  Shift In 2 : Inport  Port=4
  ASR : xbsIndex_r4/Addressable Shift Register  infer_latency=off  depth=12  initVector=[0]  en=off  dbl_ovrd=off  use_behavioral_HDL=off  use_rpm=off  block_type=addrsr
      settings: infoedit="Delay of  configurable length.  Any element  in the delay     line   can    be   addressed   and   driven    onto   the   output     port.<P><P>Hardware  notes: Implemented  using SRL16s.     If Virtex-4, Virtex-II or Spartan-3 devices are used, multiple SRLC16s are cascaded together."  xl_area=[9 0 0 18 0 0 0]  block_version=VER_STRING_GOES_HERE
  ASR1 : xbsIndex_r4/Addressable Shift Register  infer_latency=off  depth=12  initVector=[0]  en=off  dbl_ovrd=off  use_behavioral_HDL=off  use_rpm=off  block_type=addrsr
      settings: infoedit="Delay of  configurable length.  Any element  in the delay     line   can    be   addressed   and   driven    onto   the   output     port.<P><P>Hardware  notes: Implemented  using SRL16s.     If Virtex-4, Virtex-II or Spartan-3 devices are used, multiple SRLC16s are cascaded together."  xl_area=[9 0 0 18 0 0 0]  block_version=VER_STRING_GOES_HERE
  AddSub : xbsIndex_r4/AddSub  mode=Addition  use_carryin=off  use_carryout=off  en=off  latency=1  precision=User Defined  arith_type="Signed  (2's comp)"  n_bits=18  bin_pt=16  quantization="Round  (unbiased: +/- Inf)"  overflow=Saturate  dbl_ovrd=off  use_behavioral_HDL=off  pipelined=on  use_rpm=on  block_type=addsub
      settings: xl_area=[19 0 0 37 0 0 0]  block_version=VER_STRING_GOES_HERE
  Delay : xbsIndex_r4/Delay  en=off  latency=12  dbl_ovrd=off  reg_retiming=off  block_type=delay
      settings: infoedit=Hardware notes: A delay line is a chain, each link of which is an SRL16 followed by a flip-flop. If register retiming is enabled, the delay line is a chain of flip-flops.  xl_area=[9 18 0 18 0 0 0]  block_version=VER_STRING_GOES_HERE
  Delay1 : xbsIndex_r4/Delay  en=off  latency=12  dbl_ovrd=off  reg_retiming=off  block_type=delay
      settings: infoedit=Hardware notes: A delay line is a chain, each link of which is an SRL16 followed by a flip-flop. If register retiming is enabled, the delay line is a chain of flip-flops.  xl_area=[9 18 0 18 0 0 0]  block_version=VER_STRING_GOES_HERE
  Register : xbsIndex_r4/Register  init=0  rst=off  en=off  dbl_ovrd=off  block_type=register
      settings: block_version=8.2
  Register1 : xbsIndex_r4/Register  init=0  rst=off  en=off  dbl_ovrd=off  block_type=register
      settings: block_version=8.2
  Shift Out 1 : Outport
  Sum Out : Outport  Port=2
  Shift Out 2 : Outport  Port=3
  wires:
  Counter Inv/1 -> ASR1/2
  Shift In 1/1 -> ASR/1, Delay/1
  Shift In 2/1 -> Delay1/1, ASR1/1
  Counter/1 -> ASR/2
  ASR/1 -> Register/1
  ASR1/1 -> Register1/1
  AddSub/1 -> Sum Out/1
  Delay1/1 -> Shift Out 2/1
  Delay/1 -> Shift Out 1/1
  Register/1 -> AddSub/1
  Register1/1 -> AddSub/2

== system Casc_Filter_x4/DDC/DDC D/Gaussian FIR Filters/Gaussian FIR Filter1/Symmetric Data Flow/Symmetric Shift Register1 ==
  Shift In 1 : Inport
  Counter : Inport  Port=2
  Counter Inv : Inport  Port=3
  Shift In 2 : Inport  Port=4
  ASR : xbsIndex_r4/Addressable Shift Register  infer_latency=off  depth=12  initVector=[0]  en=off  dbl_ovrd=off  use_behavioral_HDL=off  use_rpm=off  block_type=addrsr
      settings: infoedit="Delay of  configurable length.  Any element  in the delay     line   can    be   addressed   and   driven    onto   the   output     port.<P><P>Hardware  notes: Implemented  using SRL16s.     If Virtex-4, Virtex-II or Spartan-3 devices are used, multiple SRLC16s are cascaded together."  xl_area=[9 0 0 18 0 0 0]  block_version=VER_STRING_GOES_HERE
  ASR1 : xbsIndex_r4/Addressable Shift Register  infer_latency=off  depth=12  initVector=[0]  en=off  dbl_ovrd=off  use_behavioral_HDL=off  use_rpm=off  block_type=addrsr
      settings: infoedit="Delay of  configurable length.  Any element  in the delay     line   can    be   addressed   and   driven    onto   the   output     port.<P><P>Hardware  notes: Implemented  using SRL16s.     If Virtex-4, Virtex-II or Spartan-3 devices are used, multiple SRLC16s are cascaded together."  xl_area=[9 0 0 18 0 0 0]  block_version=VER_STRING_GOES_HERE
  AddSub : xbsIndex_r4/AddSub  mode=Addition  use_carryin=off  use_carryout=off  en=off  latency=1  precision=User Defined  arith_type="Signed  (2's comp)"  n_bits=18  bin_pt=16  quantization="Round  (unbiased: +/- Inf)"  overflow=Saturate  dbl_ovrd=off  use_behavioral_HDL=off  pipelined=on  use_rpm=on  block_type=addsub
      settings: xl_area=[19 0 0 37 0 0 0]  block_version=VER_STRING_GOES_HERE
  Delay : xbsIndex_r4/Delay  en=off  latency=12  dbl_ovrd=off  reg_retiming=off  block_type=delay
      settings: infoedit=Hardware notes: A delay line is a chain, each link of which is an SRL16 followed by a flip-flop. If register retiming is enabled, the delay line is a chain of flip-flops.  xl_area=[9 18 0 18 0 0 0]  block_version=VER_STRING_GOES_HERE
  Delay1 : xbsIndex_r4/Delay  en=off  latency=12  dbl_ovrd=off  reg_retiming=off  block_type=delay
      settings: infoedit=Hardware notes: A delay line is a chain, each link of which is an SRL16 followed by a flip-flop. If register retiming is enabled, the delay line is a chain of flip-flops.  xl_area=[9 18 0 18 0 0 0]  block_version=VER_STRING_GOES_HERE
  Register : xbsIndex_r4/Register  init=0  rst=off  en=off  dbl_ovrd=off  block_type=register
      settings: block_version=8.2
  Register1 : xbsIndex_r4/Register  init=0  rst=off  en=off  dbl_ovrd=off  block_type=register
      settings: block_version=8.2
  Shift Out 1 : Outport
  Sum Out : Outport  Port=2
  Shift Out 2 : Outport  Port=3
  wires:
  Counter Inv/1 -> ASR1/2
  Shift In 1/1 -> ASR/1, Delay/1
  Shift In 2/1 -> Delay1/1, ASR1/1
  Counter/1 -> ASR/2
  ASR/1 -> Register/1
  ASR1/1 -> Register1/1
  AddSub/1 -> Sum Out/1
  Delay1/1 -> Shift Out 2/1
  Delay/1 -> Shift Out 1/1
  Register/1 -> AddSub/1
  Register1/1 -> AddSub/2

== system Casc_Filter_x4/DDC/DDC D/Gaussian FIR Filters/Gaussian FIR Filter1/Symmetric Data Flow/Symmetric Shift Register2 ==
  Shift In 1 : Inport
  Counter : Inport  Port=2
  Counter Inv : Inport  Port=3
  Shift In 2 : Inport  Port=4
  ASR : xbsIndex_r4/Addressable Shift Register  infer_latency=off  depth=12  initVector=[0]  en=off  dbl_ovrd=off  use_behavioral_HDL=off  use_rpm=off  block_type=addrsr
      settings: infoedit="Delay of  configurable length.  Any element  in the delay     line   can    be   addressed   and   driven    onto   the   output     port.<P><P>Hardware  notes: Implemented  using SRL16s.     If Virtex-4, Virtex-II or Spartan-3 devices are used, multiple SRLC16s are cascaded together."  xl_area=[9 0 0 18 0 0 0]  block_version=VER_STRING_GOES_HERE
  ASR1 : xbsIndex_r4/Addressable Shift Register  infer_latency=off  depth=12  initVector=[0]  en=off  dbl_ovrd=off  use_behavioral_HDL=off  use_rpm=off  block_type=addrsr
      settings: infoedit="Delay of  configurable length.  Any element  in the delay     line   can    be   addressed   and   driven    onto   the   output     port.<P><P>Hardware  notes: Implemented  using SRL16s.     If Virtex-4, Virtex-II or Spartan-3 devices are used, multiple SRLC16s are cascaded together."  xl_area=[9 0 0 18 0 0 0]  block_version=VER_STRING_GOES_HERE
  AddSub : xbsIndex_r4/AddSub  mode=Addition  use_carryin=off  use_carryout=off  en=off  latency=1  precision=User Defined  arith_type="Signed  (2's comp)"  n_bits=18  bin_pt=16  quantization="Round  (unbiased: +/- Inf)"  overflow=Saturate  dbl_ovrd=off  use_behavioral_HDL=off  pipelined=on  use_rpm=on  block_type=addsub
      settings: xl_area=[19 0 0 37 0 0 0]  block_version=VER_STRING_GOES_HERE
  Delay : xbsIndex_r4/Delay  en=off  latency=12  dbl_ovrd=off  reg_retiming=off  block_type=delay
      settings: infoedit=Hardware notes: A delay line is a chain, each link of which is an SRL16 followed by a flip-flop. If register retiming is enabled, the delay line is a chain of flip-flops.  xl_area=[9 18 0 18 0 0 0]  block_version=VER_STRING_GOES_HERE
  Delay1 : xbsIndex_r4/Delay  en=off  latency=12  dbl_ovrd=off  reg_retiming=off  block_type=delay
      settings: infoedit=Hardware notes: A delay line is a chain, each link of which is an SRL16 followed by a flip-flop. If register retiming is enabled, the delay line is a chain of flip-flops.  xl_area=[9 18 0 18 0 0 0]  block_version=VER_STRING_GOES_HERE
  Register : xbsIndex_r4/Register  init=0  rst=off  en=off  dbl_ovrd=off  block_type=register
      settings: block_version=8.2
  Register1 : xbsIndex_r4/Register  init=0  rst=off  en=off  dbl_ovrd=off  block_type=register
      settings: block_version=8.2
  Shift Out 1 : Outport
  Sum Out : Outport  Port=2
  Shift Out 2 : Outport  Port=3
  wires:
  Counter Inv/1 -> ASR1/2
  Shift In 1/1 -> ASR/1, Delay/1
  Shift In 2/1 -> Delay1/1, ASR1/1
  Counter/1 -> ASR/2
  ASR/1 -> Register/1
  ASR1/1 -> Register1/1
  AddSub/1 -> Sum Out/1
  Delay1/1 -> Shift Out 2/1
  Delay/1 -> Shift Out 1/1
  Register/1 -> AddSub/1
  Register1/1 -> AddSub/2
